simulink model "DEADZONEDYNAMIC"  (R2019a)
settings: Solver=FixedStepDiscrete  StartTime=0.0  StopTime=10.0  RelTol=1e-3
libraries: simulink x4
settings Model: Creator=saurabh  LastModifiedBy=saurabh

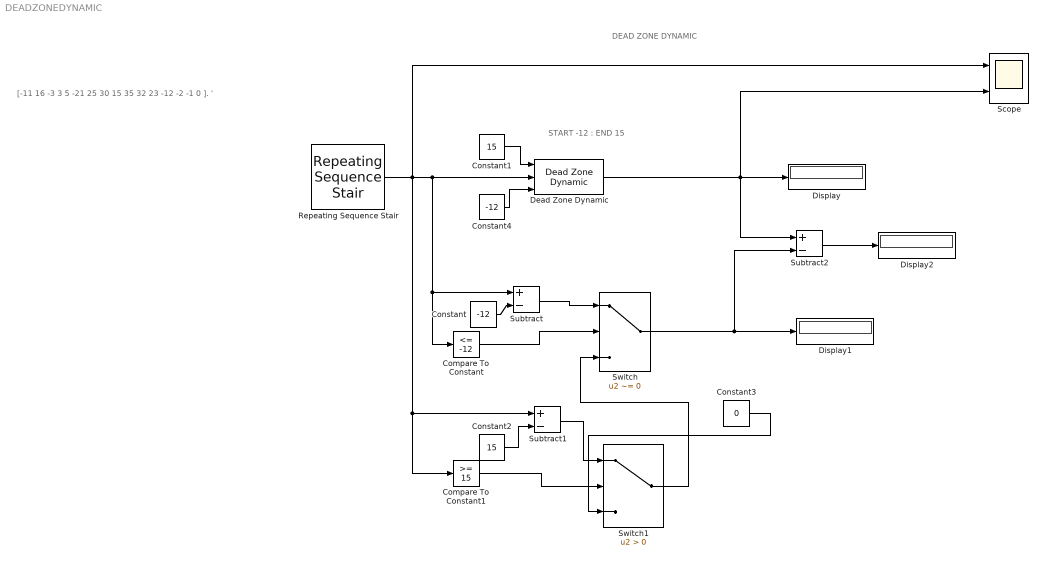
== system DEADZONEDYNAMIC ==
  note: [-11 16 -3 3 5 -21 25 30 15 35 32 23 -12 -2 -1 0 ]. '
  note: DEAD ZONE DYNAMIC
  note: START -12 : END 15
  Compare To Constant : simulink/Logic and Bit Operations/Compare To Constant  relop=<=  const=-12  OutDataTypeStr=boolean
  Compare To Constant1 : simulink/Logic and Bit Operations/Compare To Constant  relop=>=  const=15  OutDataTypeStr=boolean
  Constant : Constant  Value=-12
  Constant1 : Constant  Value=15
  Constant2 : Constant  Value=15
  Constant3 : Constant  Value=0
  Constant4 : Constant  Value=-12
  Dead Zone Dynamic : simulink/Discontinuities/Dead Zone Dynamic
      settings: SourceProductName=Simulink  SourceProductBaseCode=SL
  Display : Display
  Display1 : Display
  Display2 : Display
  Repeating Sequence Stair : simulink/Sources/Repeating Sequence Stair  OutValues="[-11 16 -3 3 5 -21 25 30 15 35 32 23 -12 -2 -1 0  ].'"  tsamp=-1  OutMin=[]  OutMax=[]  OutDataTypeStr=double  OutputDataTypeScalingMode=double  OutDataType=fixdt(0,8)  ConRadixGroup=Best Precision: Vector-wise  OutScaling=2^-12
  Scope : Scope  NumInputPorts=2
  Subtract : Sum  Inputs=+-
  Subtract1 : Sum  Inputs=+-
  Subtract2 : Sum  Inputs=+-
  Switch : Switch  Criteria=u2 ~= 0
  Switch1 : Switch  Criteria=u2 > Threshold
  wires:
  Repeating Sequence Stair/1 -> Scope/1, Subtract1/1, Compare To Constant1/1, Subtract/1, Compare To Constant/1, Dead Zone Dynamic/2
  Constant3/1 -> Switch1/3
  Subtract2/1 -> Display2/1
  Switch1/1 -> Switch/3
  Subtract1/1 -> Switch1/1
  Constant2/1 -> Subtract1/2
  Compare To Constant1/1 -> Switch1/2
  Compare To Constant/1 -> Switch/2
  Subtract/1 -> Switch/1
  Switch/1 -> Display1/1, Subtract2/2
  Constant/1 -> Subtract/2
  Dead Zone Dynamic/1 -> Scope/2, Subtract2/1, Display/1
  Constant1/1 -> Dead Zone Dynamic/1
  Constant4/1 -> Dead Zone Dynamic/3
